simulink model "I2_05_1_tr_road_sl_jpg"  (R2015a)
settings: Solver=VariableStepDiscrete  StartTime=0.0  StopTime=Inf  RelTol=1e-3
undefined symbols (not defined in the file or in its folder): gray
libraries: visionsinks x3, visiongeotforms x2, visionsources x1
settings Model: CovSFcnEnable=off  Creator=motobe  LastModifiedBy=motobe
settings OptimizationCC: ExpressionDepthLimit=2147483647
settings DebuggingCC: UnderspecifiedInitializationDetection=Classic  MergeDetectMultiDrivingBlocksExec=none  SolverPrmCheckMsg=warning  StateNameClashWarn=warning

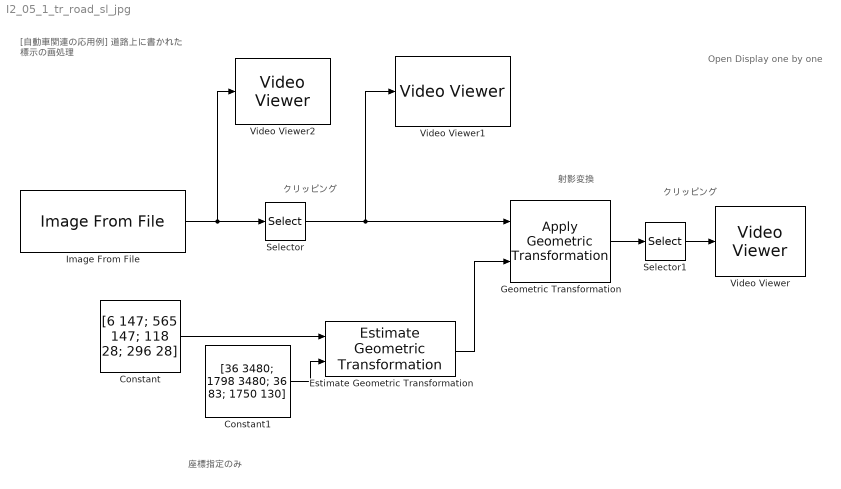
== system I2_05_1_tr_road_sl_jpg ==
  note: [自動車関連の応用例]
      |     道路上に書かれた
      |     標示の画処理
  note: Open Display one by one
  note: 座標指定のみ
  note: クリッピング
  note: クリッピング
  note: 射影変換
  Constant : Constant  Value=[6 147; 565 147; 118 28; 296 28]
  Constant1 : Constant  Value=[36 3480; 1798 3480; 36 83; 1750 130]
  Estimate Geometric Transformation : visiongeotforms/Estimate Geometric Transformation  tformType=Projective  isRandomSampling=off  algMethod=Random Sample Consensus (RANSAC)  numMethod=Specified value  isStopSampling=off  percentStop=75  distanceAlg=2.5  distanceGeo=2.5  sampleNum=500  maxSampleNum=1000  desiredConfidence=99  isRefineTForm=off  isOutputInlier=off  outDT4IntInput=Obsolete10a  outDT4IntInputActive=Single  isVarSizeAllowed=on  isReleaseMode=on
  Geometric Transformation : visiongeotforms/Apply Geometric Transformation  tformSource=Input port  tformValue=[1 0 0; 0 1 0; 0 0 1]  approxProjectiveFlag=off  errorTolerance=1.0  roiMethod=Whole input image  roiSource=Specify via dialog  roiBBox=[140 380 590 150]  roiVertice=[1 1 12 10 22 20]  inputClipFlag=off  interpolationMethod=Bilinear  fillValue=0  viewPortMethod=Specify via dialog  outputSize=[3480 5000]  outputLoc=[1 1]  outputClipFlag=off
  Image From File : visionsources/Image From File  Tag=vipblks_nd  FileName=I2_05_1_ExpTrf.jpg  imagePorts=One multidimensional signal  Ts=1  ImageDataType=double  Signed=on  WordLength=16  sdImageDataType=uint(8)  FractionLengthMode=User-defined  FractionLength=15  OutPortLabels=R|G|B
  Selector : Selector  NumberOfDimensions=3  InputPortWidth=3  IndexOptions=Index vector (dialog),Index vector (dialog),Select all  Indices=[380:530],[140:730],1  OutputSizes=1,1,1
  Selector1 : Selector  NumberOfDimensions=3  InputPortWidth=3  IndexOptions=Index vector (dialog),Index vector (dialog),Select all  Indices=[1300:3480],[1:1800],1  OutputSizes=1,1,1
  Video Viewer : visionsinks/Video Viewer  inputType=Obsolete7b  imagePorts=One multidimensional signal  useColorMap=off  colormapValue=gray(256)  specRange=off  minInputVal=0  maxInputVal=255  FigPos=[512 632 488 443]  AxisZoom=on  trueSizedOnce=off  OpenAtMdlStart=off  DefaultConfigurationName=vipscopes.VideoViewerScopeCfg
  Video Viewer1 : visionsinks/Video Viewer  inputType=Obsolete7b  imagePorts=One multidimensional signal  useColorMap=off  colormapValue=gray(256)  specRange=off  minInputVal=0  maxInputVal=255  FigPos=[450 454 410 301]  AxisZoom=on  trueSizedOnce=off  OpenAtMdlStart=off  DefaultConfigurationName=vipscopes.VideoViewerScopeCfg
  Video Viewer2 : visionsinks/Video Viewer  inputType=Obsolete7b  imagePorts=One multidimensional signal  useColorMap=off  colormapValue=gray(256)  specRange=off  minInputVal=0  maxInputVal=255  FigPos=[18 447 410 300]  AxisZoom=on  trueSizedOnce=off  OpenAtMdlStart=on  DefaultConfigurationName=vipscopes.VideoViewerScopeCfg
  wires:
  Image From File/1 -> Selector/1, Video Viewer2/1
  Geometric Transformation/1 -> Selector1/1
  Selector/1 -> Video Viewer1/1, Geometric Transformation/1
  Selector1/1 -> Video Viewer/1
  Constant/1 -> Estimate Geometric Transformation/1
  Constant1/1 -> Estimate Geometric Transformation/2
  Estimate Geometric Transformation/1 -> Geometric Transformation/2
